simulink model "Proyecto2017a"  (R2017a)
settings: Solver=VariableStepAuto  StartTime=0.0  StopTime=inf  RelTol=1e-3
values from neighbouring files (symbols this model uses):
  angle_max = 0.6108    [automatas_matlab.m]
  b_h = b_eq_h * r_h ^ 2 / R_d ^ 2    (= 28800)    [automatas_matlab.m]
  b_t = b_eq_t * r_t ^ 2 / R_w_t ^ 2    (= 27000)    [automatas_matlab.m]
  b_w_h = 30000    [automatas_matlab.m]
  ba_h = M_h * n_h * w_pos_h    (= 172800)    [automatas_matlab.m]
  ba_t = M_t * n_t * w_pos_t    (= 135000)    [automatas_matlab.m]
  g = 9.80665    [automatas_matlab.m]
  h_contenedor = 2.79    [automatas_matlab.m]
  k_bal = 10    [automatas_matlab.m]
  K_w_h = 1800000    [automatas_matlab.m]
  Ksa_h = M_h * n_h * w_pos_h^2    (= 207298.578199)    [automatas_matlab.m]
  Ksa_t = M_t * n_t * w_pos_t^2    (= 123542.570499)    [automatas_matlab.m]
  Ksia_h = M_h * w_pos_h ^ 3    (= 82894.8698367)    [automatas_matlab.m]
  Ksia_t = M_t * w_pos_t ^ 3    (= 45223.0125199)    [automatas_matlab.m]
  m_c = 50000    [automatas_matlab.m]
  M_h = (J_d + J_m_h * r_h ^ 2)/ R_d ^ 2    (= 48014.2222222)    [automatas_matlab.m]
  m_l = 65000    [automatas_matlab.m]
  M_t = m_c + (J_w_t + J_m_t * r_t ^ 2)/ R_w_t ^ 2    (= 59008)    [automatas_matlab.m]
  n_bal = 3    [automatas_matlab.m]
  R_d = 0.75    [automatas_matlab.m]
  r_h = 30    [automatas_matlab.m]
  r_t = 15    [automatas_matlab.m]
  R_w_t = 0.5    [automatas_matlab.m]
  v_max_h_load = 1.5    [automatas_matlab.m]
  v_max_h_unload = 3    [automatas_matlab.m]
  v_max_t = 4    [automatas_matlab.m]
  x_t0 = 0    [automatas_matlab.m]
  y_t0 = 45    [automatas_matlab.m]    (also in crane.m; plot_crane.m; plot_crane_test.m)
  yl0 = h_contenedor + 5    (= 7.79)    [automatas_matlab.m]
libraries: simulink x2
settings Model: Creator=elust  LastModifiedBy=laure

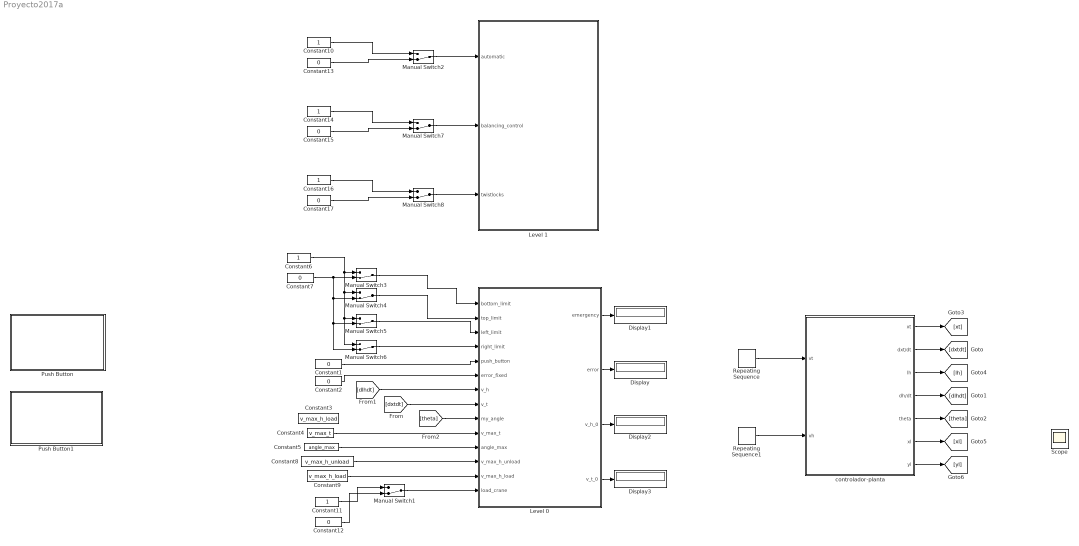
== system Proyecto2017a ==
  Constant{1..2,7,12..13,15,17} (7 alike) : Constant  Value=0
  Constant{6,10..11,14,16} (5 alike) : Constant
  Constant3 : Constant  Value=v_max_h_load
  Constant4 : Constant  Value=v_max_t
  Constant5 : Constant  Value=angle_max
  Constant8 : Constant  Value=v_max_h_unload
  Constant9 : Constant  Value=v_max_h_load
  Display{,1..3} (4 alike) : Display
  Level 0 : Stateflow chart  TreatAsAtomicUnit=on
  "Level 1 " : Stateflow chart  TreatAsAtomicUnit=on
  Manual Switch{1..8} (8 alike) : ManualSwitch  CurrentSetting=0
  Push Button : Subsystem  DialogController=hmiCreateDDGDialog  IsWebBlock=on  mask(MWDashboardBlock){webBlockId=6a905ee8-cdf0-44e2-9abf-493e9ab8f03d, webBlockType=pushbutton, ShowInLibBrwoser=on, ShowInitialText=on, HMISrcModelName=Proyecto2017a}
      mask prompts: webBlockId "WebBlock Id"; webBlockType "WebBlock Type"; HMISrcModelName "Source Model"
      mask help: SimulinkHMI:dialogs:PushButtonDialogDesc
      mask Help: helpview([docroot '/mapfiles/simulink.map'], 'hmi_push_button')
      mask Display:
      | model = bdroot(gcb);
      | if strcmp(get_param(model,'BlockDiagramType'), 'library')
      |     image([(matlabroot) '/toolbox/simulink/hmi/icons/PushButton.png']);
      | end
  Push Button1 : Subsystem  DialogController=hmiCreateDDGDialog  IsWebBlock=on  mask(MWDashboardBlock){webBlockId=faf3caf0-f0ed-4dae-b865-739de723dd10, webBlockType=pushbutton, ShowInLibBrwoser=on, ShowInitialText=on, HMISrcModelName=Proyecto2017a}
      mask prompts: webBlockId "WebBlock Id"; webBlockType "WebBlock Type"; HMISrcModelName "Source Model"
      mask help: SimulinkHMI:dialogs:PushButtonDialogDesc
      mask Help: helpview([docroot '/mapfiles/simulink.map'], 'hmi_push_button')
      mask Display:
      | model = bdroot(gcb);
      | if strcmp(get_param(model,'BlockDiagramType'), 'library')
      |     image([(matlabroot) '/toolbox/simulink/hmi/icons/PushButton.png']);
      | end
  Repeating Sequence : simulink/Sources/Repeating Sequence  rep_seq_t=[0 0.1 9.9 10]  rep_seq_y=[0 1 1 0]
  Repeating Sequence1 : simulink/Sources/Repeating Sequence  rep_seq_t=[0 1 9 10]  rep_seq_y=[0 1 1 0]
  Scope : Scope
  controlador-planta : Subsystem
  wires:
  Repeating Sequence/1 -> controlador-planta/1(vt)
  Repeating Sequence1/1 -> controlador-planta/2(vh)
  Level 0/2(error) -> Display/1
  Level 0/1(emergency) -> Display1/1
  Constant7/1 -> Manual Switch4/2, Manual Switch5/2, Manual Switch6/2, Manual Switch3/2
  Constant6/1 -> Manual Switch4/1, Manual Switch5/1, Manual Switch6/1, Manual Switch3/1
  Manual Switch3/1 -> Level 0/1(bottom_limit)
  Manual Switch4/1 -> Level 0/2(top_limit)
  Manual Switch5/1 -> Level 0/3(left_limit)
  Manual Switch6/1 -> Level 0/4(right_limit)
  Constant1/1 -> Level 0/5(push_button)
  Constant2/1 -> Level 0/6(error_fixed)
  Constant4/1 -> Level 0/10(v_max_t)
  Constant5/1 -> Level 0/11(angle_max)
  Constant8/1 -> Level 0/12(v_max_h_unload)
  Constant9/1 -> Level 0/13(v_max_h_load)
  Manual Switch1/1 -> Level 0/14(load_crane)
  Constant11/1 -> Manual Switch1/1
  Constant12/1 -> Manual Switch1/2
  controlador-planta/2(dxt/dt) -> [dxtdt]
  [dxtdt] -> Level 0/8(v_t)
  [dlhdt] -> Level 0/7(v_h)
  controlador-planta/4(dh/dt) -> [dlhdt]
  controlador-planta/5(theta) -> [theta]
  [theta] -> Level 0/9(my_angle)
  controlador-planta/1("xt ") -> [xt]
  controlador-planta/3(lh) -> [lh]
  controlador-planta/6(xl) -> [xl]
  controlador-planta/7(yl) -> [yl]
  Manual Switch2/1 -> "Level 1 "/1(automatic)
  Constant13/1 -> Manual Switch2/2
  Constant10/1 -> Manual Switch2/1
  Constant15/1 -> Manual Switch7/2
  Constant14/1 -> Manual Switch7/1
  Manual Switch7/1 -> "Level 1 "/2(balancing_control)
  Constant17/1 -> Manual Switch8/2
  Constant16/1 -> Manual Switch8/1
  Manual Switch8/1 -> "Level 1 "/3(twistlocks)
  Level 0/3(v_h_0) -> Display2/1
  Level 0/4(v_t_0) -> Display3/1

== system Proyecto2017a/Push Button ==

== system Proyecto2017a/Push Button1 ==

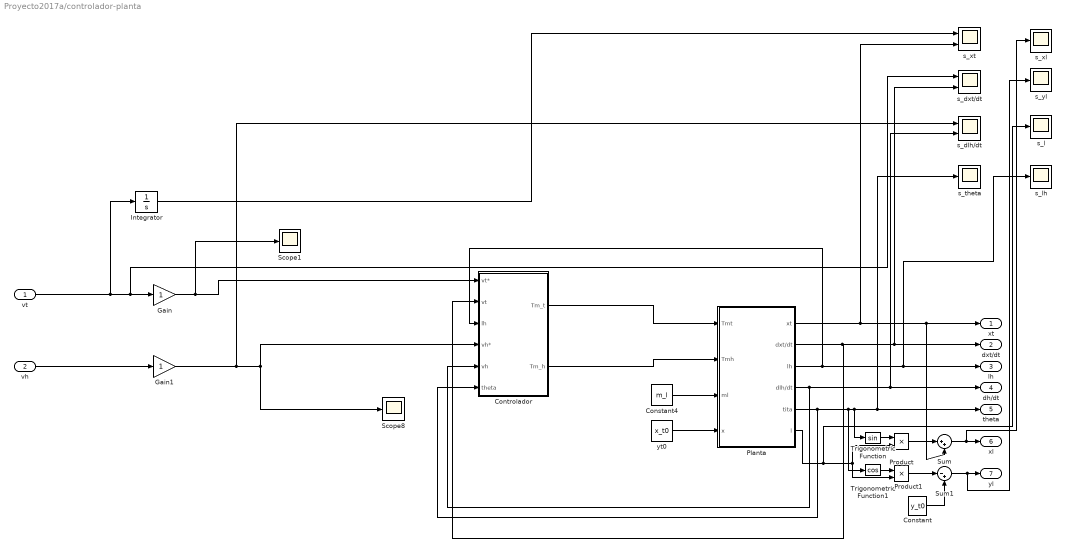
== system Proyecto2017a/controlador-planta ==
  vt : Inport
  vh : Inport  Port=2
  Constant : Constant  Value=y_t0
  Constant4 : Constant  Value=m_l
  Controlador : Subsystem
  Gain : Gain
  Gain1 : Gain
  Integrator : Integrator
  Planta : Subsystem
  Product : Product
  Product1 : Product
  Scope1 : Scope
  Scope8 : Scope
  Sum : Sum  Inputs=|++
  Sum1 : Sum  Inputs=|-+
  Trigonometric Function : Trigonometry
  Trigonometric Function1 : Trigonometry  Operator=cos
  s_dlh/dt : Scope  NumInputPorts=2
  s_dxt/dt : Scope  NumInputPorts=2
  s_l : Scope
  s_lh : Scope
  "s_theta " : Scope
  "s_xl " : Scope
  s_xt : Scope  NumInputPorts=2
  "s_yl " : Scope
  yt0 : Constant  Value=x_t0
  "xt " : Outport
  dxt/dt : Outport  Port=2
  lh : Outport  Port=3
  dh/dt : Outport  Port=4
  theta : Outport  Port=5
  xl : Outport  Port=6
  yl : Outport  Port=7
  wires:
  Gain/1 -> Controlador/1(vt*), Scope1/1
  yt0/1 -> Planta/4(x)
  Controlador/1(Tm_t) -> Planta/1(Tmt)
  Controlador/2(Tm_h) -> Planta/2(Tmh)
  Planta/5(tita) -> Trigonometric Function/1, theta/1, "s_theta "/1, Trigonometric Function1/1, Controlador/6(theta)
  Planta/4(dlh/dt) -> dh/dt/1, s_dlh/dt/2, Controlador/5(vh)
  Constant4/1 -> Planta/3(ml)
  Planta/2(dxt/dt) -> Controlador/2(vt), s_dxt/dt/2, dxt/dt/1
  Planta/3(lh) -> s_lh/1, lh/1, Controlador/3(lh)
  vt/1 -> Integrator/1, s_dxt/dt/1, Gain/1
  vh/1 -> Gain1/1
  Gain1/1 -> s_dlh/dt/1, Controlador/4(vh*), Scope8/1
  Planta/1(xt) -> s_xt/2, Sum/2, "xt "/1
  Planta/6(l) -> s_l/1, Product/2, Product1/2
  Trigonometric Function1/1 -> Product1/1
  Trigonometric Function/1 -> Product/1
  Sum/1 -> "s_xl "/1, xl/1
  Product/1 -> Sum/1
  Product1/1 -> Sum1/1
  Constant/1 -> Sum1/2
  Integrator/1 -> s_xt/1
  Sum1/1 -> "s_yl "/1, yl/1

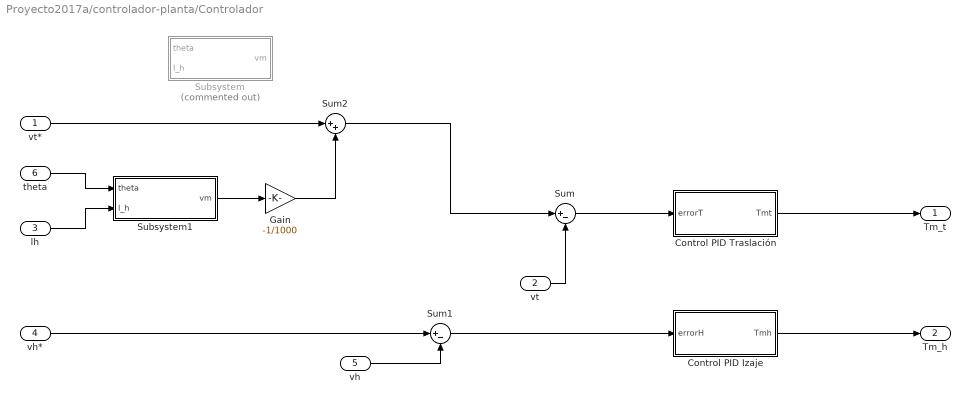
== system Proyecto2017a/controlador-planta/Controlador ==
  vt* : Inport
  vt : Inport  Port=2
  lh : Inport  Port=3
  vh* : Inport  Port=4
  vh : Inport  Port=5
  theta : Inport  Port=6
  Control PID Izaje : Subsystem
  "Control PID Traslación " : Subsystem
  Gain : Gain  Gain=-1/1000
  Subsystem : Subsystem  Commented=on
  Subsystem1 : Subsystem
  Sum : Sum  Inputs=|+-
  Sum1 : Sum  Inputs=|+-
  Sum2 : Sum  Inputs=|++
  Tm_t : Outport
  Tm_h : Outport  Port=2
  wires:
  vt/1 -> Sum/2
  lh/1 -> Subsystem1/2(I_h)
  theta/1 -> Subsystem1/1(theta)
  Subsystem1/1(vm) -> Gain/1
  vt*/1 -> Sum2/1
  "Control PID Traslación "/1(Tmt) -> Tm_t/1
  vh*/1 -> Sum1/1
  Sum2/1 -> Sum/1
  Control PID Izaje/1(Tmh) -> Tm_h/1
  vh/1 -> Sum1/2
  Sum1/1 -> Control PID Izaje/1(errorH)
  Sum/1 -> "Control PID Traslación "/1(errorT)
  Gain/1 -> Sum2/2

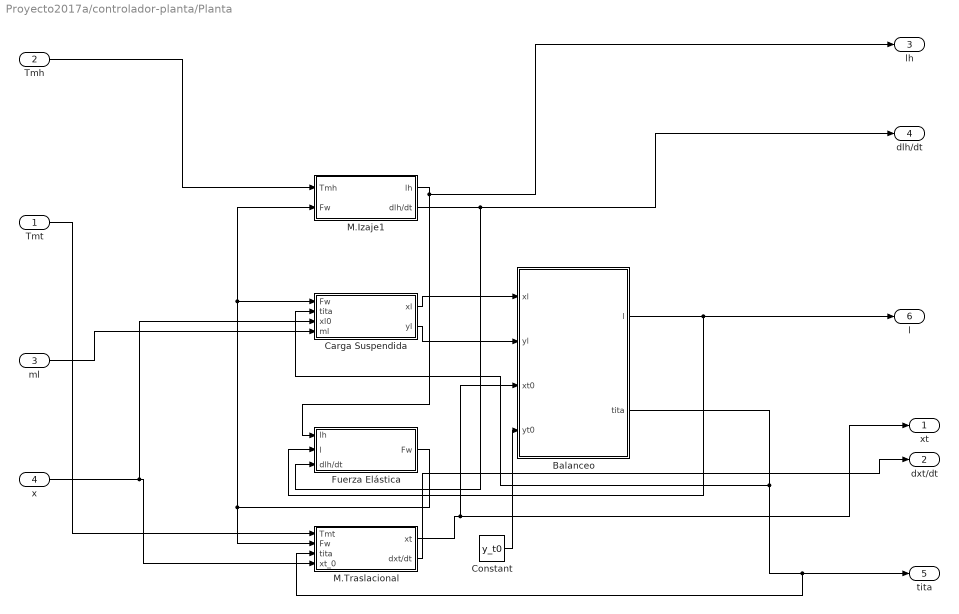
== system Proyecto2017a/controlador-planta/Planta ==
  Tmt : Inport
  Tmh : Inport  Port=2
  ml : Inport  Port=3
  x : Inport  Port=4
  Balanceo : MATLAB Function  TreatAsAtomicUnit=on
  Carga Suspendida : Subsystem
  Constant : Constant  Value=y_t0
  Fuerza Elástica : Subsystem
  M.Izaje1 : Subsystem
  M.Traslacional : Subsystem
  xt : Outport
  dxt/dt : Outport  Port=2
  lh : Outport  Port=3
  dlh/dt : Outport  Port=4
  tita : Outport  Port=5
  l : Outport  Port=6
  wires:
  Balanceo/2(tita) -> Carga Suspendida/2(tita), M.Traslacional/3(tita), tita/1
  Balanceo/1(l) -> Fuerza Elástica/2(l), l/1
  M.Izaje1/2(dlh/dt) -> Fuerza Elástica/3(dlh/dt), dlh/dt/1
  Fuerza Elástica/1(Fw) -> M.Traslacional/2(Fw), Carga Suspendida/1(Fw), M.Izaje1/2(Fw)
  x/1 -> Carga Suspendida/3(xl0), M.Traslacional/4(xt_0)
  ml/1 -> Carga Suspendida/4(ml)
  M.Izaje1/1(lh) -> lh/1, Fuerza Elástica/1(lh)
  Tmh/1 -> M.Izaje1/1(Tmh)
  Tmt/1 -> M.Traslacional/1("Tmt ")
  Carga Suspendida/1(xl) -> Balanceo/1(xl)
  Carga Suspendida/2(yl) -> Balanceo/2(yl)
  M.Traslacional/1(xt) -> Balanceo/3(xt0), xt/1
  M.Traslacional/2(dxt/dt) -> dxt/dt/1
  Constant/1 -> Balanceo/4(yt0)

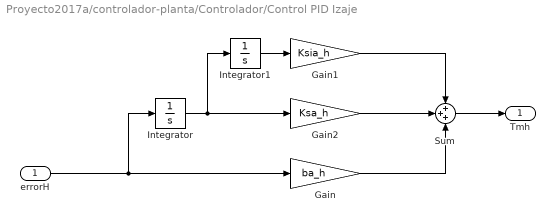
== system Proyecto2017a/controlador-planta/Controlador/Control PID Izaje ==
  errorH : Inport
  Gain : Gain  Gain=ba_h
  Gain1 : Gain  Gain=Ksia_h
  Gain2 : Gain  Gain=Ksa_h
  Integrator : Integrator
  Integrator1 : Integrator
  Sum : Sum  Inputs=+++
  Tmh : Outport
  wires:
  Integrator1/1 -> Gain1/1
  errorH/1 -> Integrator/1, Gain/1
  Gain2/1 -> Sum/2
  Gain1/1 -> Sum/1
  Gain/1 -> Sum/3
  Sum/1 -> Tmh/1
  Integrator/1 -> Integrator1/1, Gain2/1

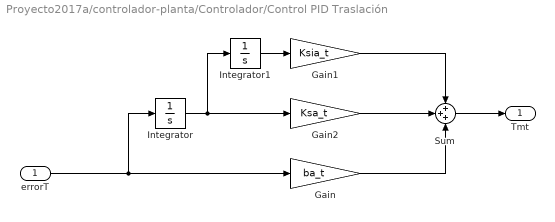
== system Proyecto2017a/controlador-planta/Controlador/Control PID Traslación  ==
  errorT : Inport
  Gain : Gain  Gain=ba_t
  Gain1 : Gain  Gain=Ksia_t
  Gain2 : Gain  Gain=Ksa_t
  Integrator : Integrator
  Integrator1 : Integrator
  Sum : Sum  Inputs=+++
  Tmt : Outport
  wires:
  Integrator1/1 -> Gain1/1
  errorT/1 -> Integrator/1, Gain/1
  Gain2/1 -> Sum/2
  Gain1/1 -> Sum/1
  Gain/1 -> Sum/3
  Sum/1 -> Tmt/1
  Integrator/1 -> Integrator1/1, Gain2/1

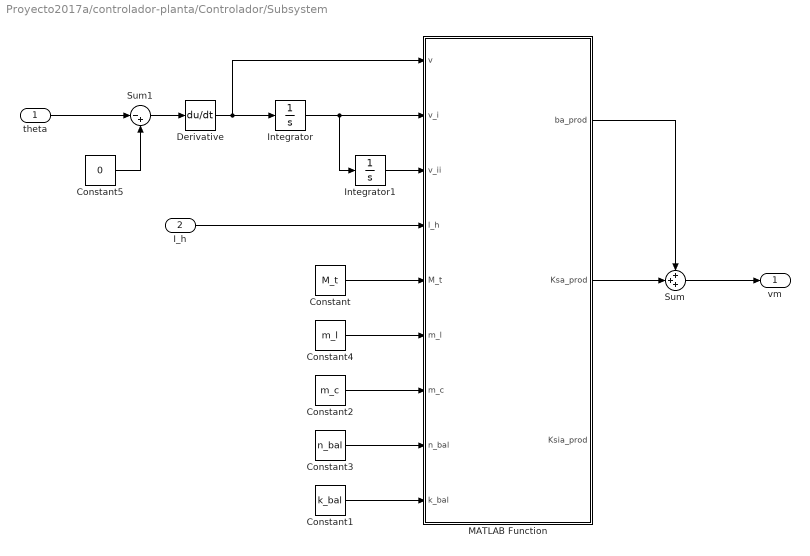
== system Proyecto2017a/controlador-planta/Controlador/Subsystem ==
  theta : Inport
  I_h : Inport  Port=2
  Constant : Constant  Value=M_t
  Constant1 : Constant  Value=k_bal
  Constant2 : Constant  Value=m_c
  Constant3 : Constant  Value=n_bal
  Constant4 : Constant  Value=m_l
  Constant5 : Constant  Value=0
  Derivative : Derivative
  Integrator : Integrator
  Integrator1 : Integrator
  MATLAB Function : MATLAB Function  TreatAsAtomicUnit=on
  Sum : Sum  Inputs=+++
  Sum1 : Sum  Inputs=|-+
  vm : Outport
  wires:
  MATLAB Function/1(ba_prod) -> Sum/1
  I_h/1 -> MATLAB Function/4(l_h)
  MATLAB Function/2(Ksa_prod) -> Sum/2
  theta/1 -> Sum1/1
  Integrator/1 -> Integrator1/1, MATLAB Function/2(v_i)
  Sum/1 -> vm/1
  Integrator1/1 -> MATLAB Function/3(v_ii)
  Constant/1 -> MATLAB Function/5(M_t)
  Constant2/1 -> MATLAB Function/7(m_c)
  Constant3/1 -> MATLAB Function/8(n_bal)
  Constant1/1 -> MATLAB Function/9(k_bal)
  Constant4/1 -> MATLAB Function/6(m_l)
  Constant5/1 -> Sum1/2
  Sum1/1 -> Derivative/1
  Derivative/1 -> MATLAB Function/1(v), Integrator/1

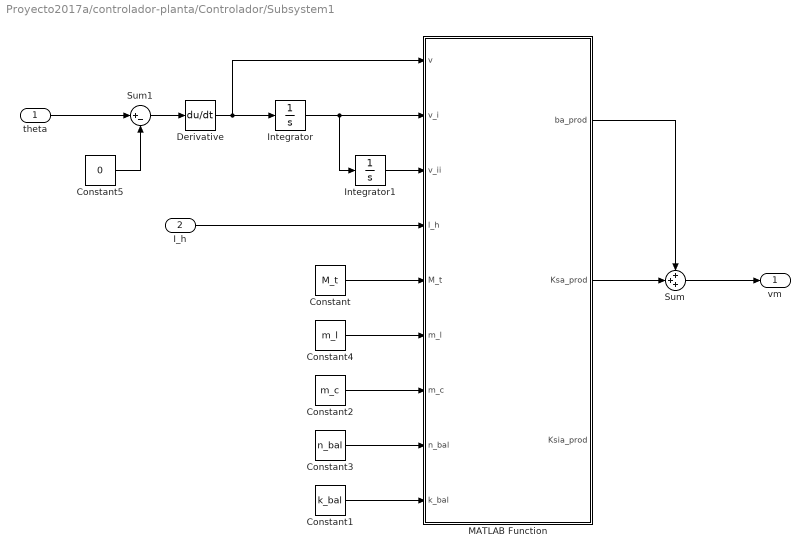
== system Proyecto2017a/controlador-planta/Controlador/Subsystem1 ==
  theta : Inport
  I_h : Inport  Port=2
  Constant : Constant  Value=M_t
  Constant1 : Constant  Value=k_bal
  Constant2 : Constant  Value=m_c
  Constant3 : Constant  Value=n_bal
  Constant4 : Constant  Value=m_l
  Constant5 : Constant  Value=0
  Derivative : Derivative
  Integrator : Integrator
  Integrator1 : Integrator
  MATLAB Function : MATLAB Function  TreatAsAtomicUnit=on
  Sum : Sum  Inputs=+++
  Sum1 : Sum  Inputs=|+-
  vm : Outport
  wires:
  MATLAB Function/1(ba_prod) -> Sum/1
  I_h/1 -> MATLAB Function/4(l_h)
  MATLAB Function/2(Ksa_prod) -> Sum/2
  theta/1 -> Sum1/1
  Integrator/1 -> Integrator1/1, MATLAB Function/2(v_i)
  Sum/1 -> vm/1
  Integrator1/1 -> MATLAB Function/3(v_ii)
  Constant/1 -> MATLAB Function/5(M_t)
  Constant2/1 -> MATLAB Function/7(m_c)
  Constant3/1 -> MATLAB Function/8(n_bal)
  Constant1/1 -> MATLAB Function/9(k_bal)
  Constant4/1 -> MATLAB Function/6(m_l)
  Constant5/1 -> Sum1/2
  Sum1/1 -> Derivative/1
  Derivative/1 -> MATLAB Function/1(v), Integrator/1

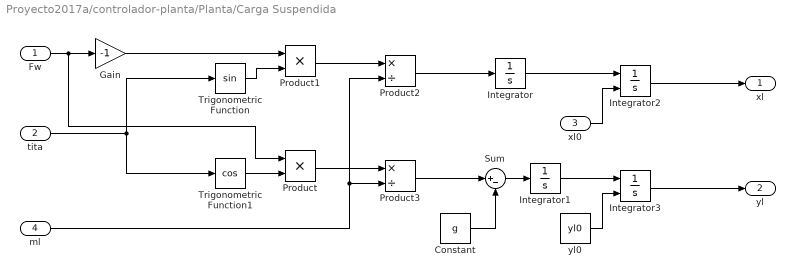
== system Proyecto2017a/controlador-planta/Planta/Carga Suspendida ==
  Fw : Inport
  tita : Inport  Port=2
  xl0 : Inport  Port=3
  ml : Inport  Port=4
  Constant : Constant  Value=g
  Gain : Gain  Gain=-1
  Integrator : Integrator
  Integrator1 : Integrator
  Integrator2 : Integrator  InitialConditionSource=external
  Integrator3 : Integrator  InitialConditionSource=external
  Product : Product
  Product1 : Product
  Product2 : Product  Inputs=*/
  Product3 : Product  Inputs=*/
  Sum : Sum  Inputs=|+-
  Trigonometric Function : Trigonometry
  Trigonometric Function1 : Trigonometry  Operator=cos
  yl0 : Constant  Value=yl0
  xl : Outport
  yl : Outport  Port=2
  wires:
  tita/1 -> Trigonometric Function/1, Trigonometric Function1/1
  Constant/1 -> Sum/2
  Trigonometric Function1/1 -> Product/2
  Fw/1 -> Product/1, Gain/1
  Trigonometric Function/1 -> Product1/2
  Sum/1 -> Integrator1/1
  Integrator/1 -> Integrator2/1
  Integrator1/1 -> Integrator3/1
  yl0/1 -> Integrator3/2
  xl0/1 -> Integrator2/2
  Integrator2/1 -> xl/1
  Integrator3/1 -> yl/1
  Product/1 -> Product3/1
  Product1/1 -> Product2/1
  ml/1 -> Product2/2, Product3/2
  Product2/1 -> Integrator/1
  Product3/1 -> Sum/1
  Gain/1 -> Product1/1

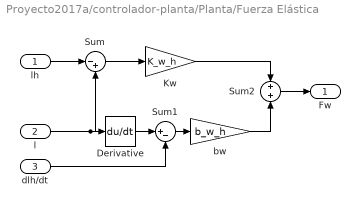
== system Proyecto2017a/controlador-planta/Planta/Fuerza Elástica ==
  lh : Inport
  l : Inport  Port=2
  dlh/dt : Inport  Port=3
  Derivative : Derivative
  Kw : Gain  Gain=K_w_h
  Sum : Sum  Inputs=|-+
  Sum1 : Sum  Inputs=|+-
  Sum2 : Sum
  bw : Gain  Gain=b_w_h
  Fw : Outport
  wires:
  l/1 -> Sum/2, Derivative/1
  lh/1 -> Sum/1
  Sum/1 -> Kw/1
  Derivative/1 -> Sum1/1
  dlh/dt/1 -> Sum1/2
  Sum1/1 -> bw/1
  Sum2/1 -> Fw/1
  Kw/1 -> Sum2/1
  bw/1 -> Sum2/2

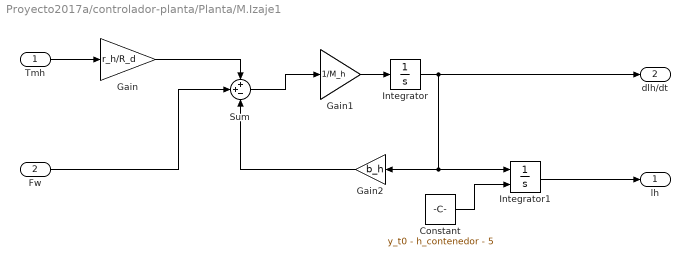
== system Proyecto2017a/controlador-planta/Planta/M.Izaje1 ==
  Tmh : Inport
  Fw : Inport  Port=2
  Constant : Constant  Value=y_t0 - h_contenedor - 5
  Gain : Gain  Gain=r_h/R_d
  Gain1 : Gain  Gain=1/M_h
  Gain2 : Gain  Gain=b_h
  Integrator : Integrator
  Integrator1 : Integrator  InitialConditionSource=external
  Sum : Sum  Inputs=++-
  lh : Outport
  dlh/dt : Outport  Port=2
  wires:
  Tmh/1 -> Gain/1
  Gain/1 -> Sum/1
  Sum/1 -> Gain1/1
  Gain1/1 -> Integrator/1
  Integrator/1 -> dlh/dt/1, Integrator1/1, Gain2/1
  Gain2/1 -> Sum/3
  Fw/1 -> Sum/2
  Constant/1 -> Integrator1/2
  Integrator1/1 -> lh/1

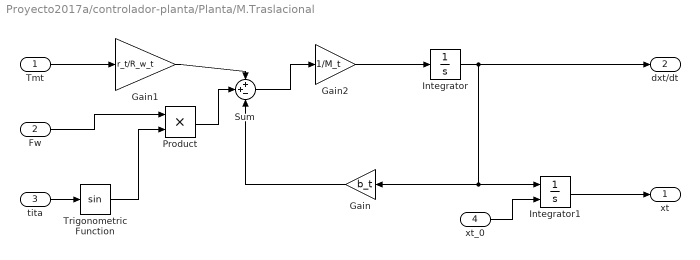
== system Proyecto2017a/controlador-planta/Planta/M.Traslacional ==
  "Tmt " : Inport
  Fw : Inport  Port=2
  tita : Inport  Port=3
  xt_0 : Inport  Port=4
  Gain : Gain  Gain=b_t
  Gain1 : Gain  Gain=r_t/R_w_t
  Gain2 : Gain  Gain=1/M_t
  Integrator : Integrator
  Integrator1 : Integrator  InitialConditionSource=external
  Product : Product
  Sum : Sum  Inputs=++-
  Trigonometric Function : Trigonometry
  xt : Outport
  dxt/dt : Outport  Port=2
  wires:
  Gain2/1 -> Integrator/1
  Trigonometric Function/1 -> Product/2
  tita/1 -> Trigonometric Function/1
  Integrator/1 -> dxt/dt/1, Integrator1/1, Gain/1
  Gain/1 -> Sum/3
  Fw/1 -> Product/1
  Product/1 -> Sum/2
  Sum/1 -> Gain2/1
  Gain1/1 -> Sum/1
  xt_0/1 -> Integrator1/2
  "Tmt "/1 -> Gain1/1
  Integrator1/1 -> xt/1

== matlab function Proyecto2017a/controlador-planta/Controlador/Subsystem/MATLAB Function ==
  data: ba_prod output; Ksa_prod output; Ksia_prod output; v input; v_i input; v_ii input; l_h input; M_t input; m_l input; m_c input; n_bal input; k_bal input
function [ba_prod, Ksa_prod, Ksia_prod] = fcn(v, v_i, v_ii, l_h, M_t, m_l, m_c, n_bal, k_bal)


poles = sqrt(complex((-M_t)/ ((M_t + m_l)* l_h)));
w_n = abs(poles(1))

w_pos = k_bal * w_n;

J_eq = - (M_t + m_l) * l_h /(m_c + m_l);



ba = J_eq * n_bal * w_pos;
Ksa = J_eq * n_bal * w_pos ^ 2;
Ksia = J_eq * w_pos ^ 3;


ba_prod = ba * v;
Ksa_prod = Ksa * v_i;
Ksia_prod = Ksia * v_ii;



end

== stateflow chart Proyecto2017a/Level 0 ==
  state Level0
    state Emergency_limit_switch_horizontal
      entry:
      emergency = 1;
      if (right_limit == 1)
      error = 1;
      else
      error = 2;
      end
    state Normal
      entry:
      if (load_crane == 0)
      v_max_h = v_max_h_unload
      else
      v_max_h = v_max_h_load
      end
      emergency = 0;
      error = 0;
    state Emergency_limit_switch_vertical
      entry:
      emergency = 1;
      if (bottom_limit == 1)
      error = 3;
      else
      error = 4;
      end
    state Emergency_overspeed
      entry:
      emergency = 1;
      error = 5;
    state Emergency_button
      entry:
      emergency = 1;
      error = 6;
    state Emergency_angle
      entry:
      emergency = 1;
      error = 7;
    Normal -> Emergency_limit_switch_horizontal [order 1] : [(right_limit == 1)||(left_limit == 1)]
    (default) -> Normal
    Normal -> Emergency_limit_switch_vertical [order 2] : [(top_limit == 1) || (bottom_limit == 1)]
    Normal -> Emergency_overspeed [order 4] : [ (v_t > abs(v_max_t)) || (v_h > abs(v_max_h))]
    Normal -> Emergency_angle [order 5] : [my_angle > angle_max]
    Normal -> Emergency_button [order 3] : [push_button == 1]
  state Emergency
    state emergency_handler
      during:
      disp('EMERGENCY')
      [v_t_0, v_h_0] = handleError(error)
    state end_emergency
      entry:
      emergency = 0
      error = 0
    (default) -> emergency_handler
    emergency_handler -> end_emergency : [error_fixed == 1]
  (default) -> Level0
  Level0 -> Emergency : [emergency == 1]
  Emergency -> Level0 : [emergency == 0]
  data: my_error function_input; v_t_o function_output; v_h_o function_output; emergency output; bottom_limit input; top_limit input; left_limit input; right_limit input; push_button input; error_fixed input; error output; v_h input; v_t input; my_angle input; v_max_t input double; angle_max input double; v_max_h_unload input; v_max_h_load input; v_max_h local double; load_crane input; v_h_0 output; v_t_0 output
  function [v_t_o, v_h_o] = handleError(my_error):
    | function [v_t_o, v_h_o] = handleError(my_error)
    | v_t_o = v_t;
    | v_h_o = v_h;
    | if (my_error == 1) || (my_error == 2) % Right and left
    |     v_t_o = 0;
    | elseif (my_error == 3) || (my_error == 4) % Botton and top
    |     v_h_o = 0;
    | elseif (my_error == 5) % Overspeed
    |     v_t_o = 0;
    |     v_h_o = 0;
    | elseif (my_error == 6) % Emergency button
    |     v_t_o = 0;
    |     v_h_o = 0;
    | elseif (my_error == 7) % Emergency angle
    |     v_h_o = 0;
    |     v_t_o = 0;
    | end
    | end

== matlab function Proyecto2017a/controlador-planta/Planta/Balanceo ==
  data: xl input; l output; yl input; xt0 input; yt0 input; tita output
function [l,tita] = fcn(xl,yl,xt0,yt0)

deltax = (xl - xt0);
deltay = -(yl - yt0);


l = sqrt((deltax ^ 2) + (deltay ^ 2));

tita = atan2(deltax, deltay);

end

== matlab function Proyecto2017a/controlador-planta/Controlador/Subsystem1/MATLAB Function ==
  data: ba_prod output; Ksa_prod output; Ksia_prod output; v input; v_i input; v_ii input; l_h input; M_t input; m_l input; m_c input; n_bal input; k_bal input
function [ba_prod, Ksa_prod, Ksia_prod] = fcn(v, v_i, v_ii, l_h, M_t, m_l, m_c, n_bal, k_bal)


poles = sqrt(complex(-M_t * 9.8/ ((M_t + m_l)* l_h)));
w_n = abs(poles(1));

w_pos = k_bal * w_n;

J_eq = - (M_t + m_l) * l_h /(m_c + m_l);

ba = J_eq * n_bal * w_pos;
Ksa = J_eq * n_bal * w_pos ^ 2;
Ksia = J_eq * w_pos ^ 3;


ba_prod = ba * v;
Ksa_prod = Ksa * v_i;
Ksia_prod = Ksia * v_ii;



end

== stateflow chart Proyecto2017a/Level 1  ==
  state Level1
    state Start [parallel]
      settings: executionOrder=1
      state Manual
        entry:
        during:
      state Automatico
        entry:
        during:
      (default) -> Manual
      Manual -> Automatico : [automatic == 1]
      Automatico -> Manual : [automatic == 0]
    state Spreader [parallel]
      settings: executionOrder=2
      state Charged
      state Unchaged
      (default) -> Charged
      Charged -> Unchaged : [twistlocks == 0]
      Unchaged -> Charged : [twistlocks == 1]
    state Balancing_Control [parallel]
      settings: executionOrder=3
      state Activated
      state Disactivated
      (default) -> Activated
      Activated -> Disactivated : [balancing_control == 0]
      Disactivated -> Activated : [balancing_control == 1]
  note: ?
  (default) -> Level1
  data: automatic input; balancing_control input; twistlocks input
